simulink model "VerificaLQR_27042026"  (R2025b)
settings: Solver=VariableStepAuto  StartTime=0.0  StopTime=10.0  RelTol=1e-3
values from neighbouring files (symbols this model uses):
  A = double(subs(A_sym, [x; u], [x_star; u_star]))    [Esame_27042026.m]
  B = double(subs(B_sym, [x; u], [x_star; u_star]))    [Esame_27042026.m]
  C = eye(n)    [Esame_27042026.m]
  C_LQR = C_inseguimento_EIG    [Esame_27042026.m]
  D = zeros(n, m)    [Esame_27042026.m]
  K_LQR_i = K_LQR(:, n+1:end)    [Esame_27042026.m]
  K_LQR_x = K_LQR(:, 1:n)    [Esame_27042026.m]
undefined symbols (not defined in the file or in its folder): x0_LQR, x_ref_lqr
settings Model: Creator=salvo  LastModifiedBy=salvo

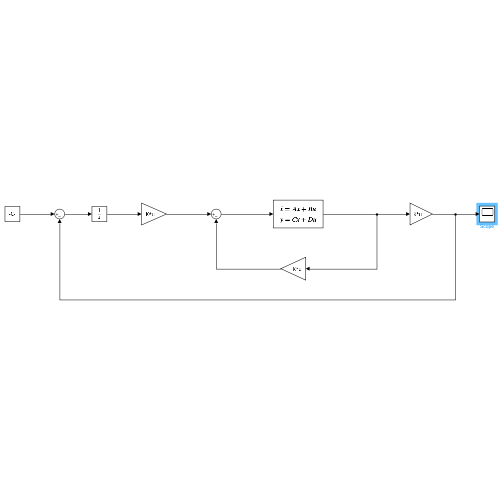
[thumbnail: Simulink's stored preview of the top-level diagram]
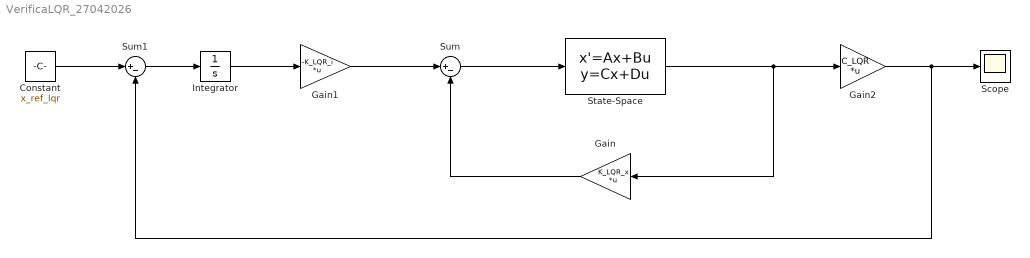
== system VerificaLQR_27042026 ==
  Constant : Constant  Value=x_ref_lqr
  Gain : Gain  Gain=K_LQR_x  Multiplication=Matrix(K*u)
  Gain1 : Gain  Gain=-K_LQR_i  Multiplication=Matrix(K*u)
  Gain2 : Gain  Gain=C_LQR  Multiplication=Matrix(K*u)
  Integrator : Integrator
  Scope : Scope
      settings: ActiveDisplayYMinimum=-35.225981398916929  ActiveDisplayYMaximum=52.416268897192225
  State-Space : StateSpace  A=A  B=B  C=C  D=D  InitialCondition=x0_LQR
  Sum : Sum  Inputs=|+-
  Sum1 : Sum  Inputs=|+-
  wires:
  State-Space/1 -> Gain/1, Gain2/1
  Sum/1 -> State-Space/1
  Gain/1 -> Sum/2
  Gain1/1 -> Sum/1
  Constant/1 -> Sum1/1
  Sum1/1 -> Integrator/1
  Integrator/1 -> Gain1/1
  Gain2/1 -> Sum1/2, Scope/1
